simulink model "ACS_1"  (Simulink 7.6)
settings: Solver=ode45  StartTime=0.0  StopTime=1  RelTol=1e-3
settings Model: Creator=Vano  LastModifiedBy=Vano

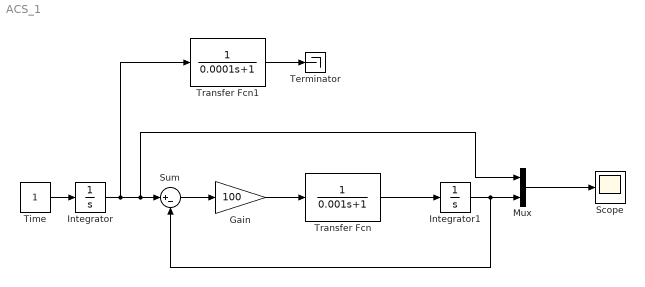
== system ACS_1 ==
  Gain : Gain  Gain=100
  Integrator : Integrator
  Integrator1 : Integrator
  Mux : Mux  Inputs=2
  Scope : Scope
  Sum : Sum  Inputs=|+-
  Terminator : Terminator
  Time : Constant
  Transfer Fcn : TransferFcn  Denominator=[0.001 1]
  Transfer Fcn1 : TransferFcn  Denominator=[0.0001 1]
  wires:
  Transfer Fcn/1 -> Integrator1/1
  Time/1 -> Integrator/1
  Integrator/1 -> Sum/1, Mux/1, Transfer Fcn1/1
  Sum/1 -> Gain/1
  Gain/1 -> Transfer Fcn/1
  Integrator1/1 -> Mux/2, Sum/2
  Mux/1 -> Scope/1
  Transfer Fcn1/1 -> Terminator/1
